simulink model "Proj_SW"  (R2020a)
settings: Solver=VariableStepAuto  StartTime=0.0  StopTime=10.0  RelTol=1e-3
undefined symbols (not defined in the file): T
settings Model: Creator=jguil  LastModifiedBy=jguil

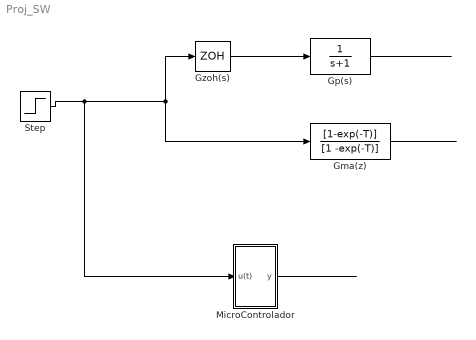
== system Proj_SW ==
  Gma(z) : DiscreteTransferFcn  Numerator=[1-exp(-T)]  Denominator=[1 -exp(-T)]
  Gp(s) : TransferFcn  Denominator=[1 1]
  Gzoh(s) : ZeroOrderHold  SampleTime=-1
  MicroControlador : Subsystem
  Step : Step  SampleTime=0
  wires:
  Gzoh(s)/1 -> Gp(s)/1
  Step/1 -> MicroControlador/1(u(t)), Gma(z)/1, Gzoh(s)/1
  Gma(z)/1 -> ?
  Gp(s)/1 -> ?
  MicroControlador/1(y) -> ?

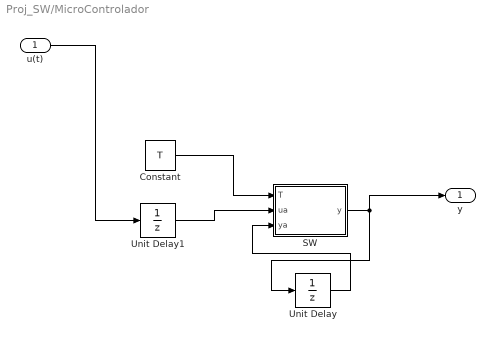
== system Proj_SW/MicroControlador ==
  u(t) : Inport
  Constant : Constant  Value=T
  SW : MATLAB Function  TreatAsAtomicUnit=on
  Unit Delay : UnitDelay  SampleTime=-1  HasFrameUpgradeWarning=on
  Unit Delay1 : UnitDelay  SampleTime=T  HasFrameUpgradeWarning=on
  y : Outport
  wires:
  Unit Delay/1 -> SW/3(ya)
  Unit Delay1/1 -> SW/2(ua)
  SW/1(y) -> y/1, Unit Delay/1
  Constant/1 -> SW/1(T)
  u(t)/1 -> Unit Delay1/1

== matlab function Proj_SW/MicroControlador/SW ==
  data: T input; y output; ua input; ya input
function y = ModeloSW(T,ua,ya)

a = 1-exp(-T);
b=exp(-T);

y = a*ua+b*ya;
